simulink model "chan_snap_v3"  (R2012b)
settings: Solver=ode45  StartTime=0.0  StopTime=10000  RelTol=1e-3
undefined symbols (not defined in the file): pfb_coeff_gen_calc, xlipgetpartsetting
libraries: xbsIndex_r4 x7452, casper_library_misc x131, casper_library_flow_control x107, casper_library_delays x40, xps_library x8
(part 3 of 84)

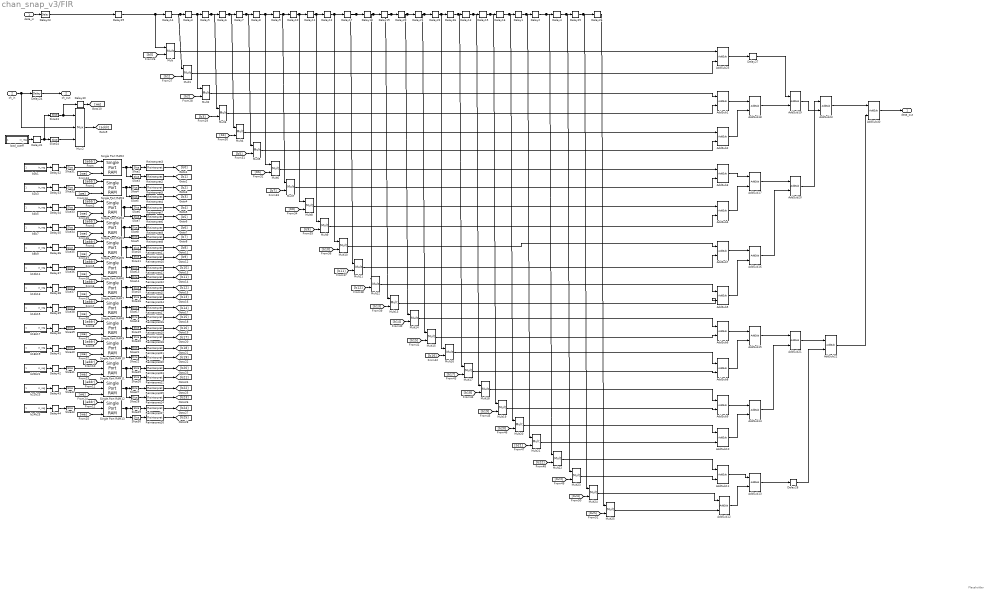
== system chan_snap_v3/FIR ==
  note: Placeholder
  data_in : Inport
  ch_in : Inport  Port=2
  AddSub{1..23,25} (24 alike) : xbsIndex_r4/AddSub  mode=Addition  use_carryin=off  use_carryout=off  en=off  latency=3  precision=Full  arith_type="Signed  (2's comp)"  n_bits=16  bin_pt=15  quantization=Truncate  overflow=Wrap  dbl_ovrd=off  use_behavioral_HDL=off  hw_selection=DSP48  pipelined=on  block_type=addsub
  AddSub40 : xbsIndex_r4/AddSub  mode=Addition  use_carryin=off  use_carryout=off  en=off  latency=3  precision=User Defined  arith_type="Signed  (2's comp)"  n_bits=12  bin_pt=9  quantization=Truncate  overflow=Wrap  dbl_ovrd=off  use_behavioral_HDL=off  hw_selection=DSP48  pipelined=on  block_type=addsub
  Delay{1..22,25..26,46} (25 alike) : xbsIndex_r4/Delay  rst=off  infoeditControl=Selection of Reset will increase slice count due to use of real FFs and instead of SRLs  en=off  latency=256  dbl_ovrd=off  reg_retiming=off  block_type=delay
      settings: block_version=11.4
  Delay{23,30..44} (16 alike) : xbsIndex_r4/Delay  rst=off  infoeditControl=Selection of Reset will increase slice count due to use of real FFs and instead of SRLs  en=off  latency=1  dbl_ovrd=off  reg_retiming=off  block_type=delay
      settings: block_version=11.4
  Delay24 : xbsIndex_r4/Delay  rst=off  infoeditControl=Selection of Reset will increase slice count due to use of real FFs and instead of SRLs  en=off  latency=24  dbl_ovrd=off  reg_retiming=off  block_type=delay
      settings: block_version=11.4
  Delay27 : xbsIndex_r4/Delay  rst=off  infoeditControl=Selection of Reset will increase slice count due to use of real FFs and instead of SRLs  en=off  latency=3  dbl_ovrd=off  reg_retiming=off  block_type=delay
      settings: block_version=11.4
  Delay28 : xbsIndex_r4/Delay  rst=off  infoeditControl=Selection of Reset will increase slice count due to use of real FFs and instead of SRLs  en=off  latency=3  dbl_ovrd=off  reg_retiming=off  block_type=delay
      settings: block_version=11.4
  Delay29 : xbsIndex_r4/Delay  rst=off  infoeditControl=Selection of Reset will increase slice count due to use of real FFs and instead of SRLs  en=off  latency=3  dbl_ovrd=off  reg_retiming=off  block_type=delay
      settings: block_version=11.4
  Mult{,1..25} (26 alike) : xbsIndex_r4/Mult  precision=Full  arith_type="Signed  (2's comp)"  n_bits=16  bin_pt=14  quantization=Truncate  overflow=Wrap  en=off  latency=5  dbl_ovrd=off  use_behavioral_HDL=off  opt=Speed  use_embedded=on  optimum_pipeline=on  pipeline=on  use_rpm=on  placement_style=Triangular  block_type=mult
      settings: block_version=11.4
  Mux2 : xbsIndex_r4/Mux  inputs=2  en=off  latency=1  precision=Full  arith_type=Unsigned  n_bits=16  bin_pt=14  quantization=Truncate  overflow=Wrap  dbl_ovrd=off  block_type=mux
      settings: block_version=11.4
  Reinterpret{2..27} (26 alike) : xbsIndex_r4/Reinterpret  force_arith_type=on  arith_type="Signed  (2's comp)"  force_bin_pt=on  bin_pt=11  block_type=reinterpret
      settings: infoedit="Changes signal type without altering the binary representation.   You can changed the signal between signed and unsigned, and relocate the binary point.<br><br>Hardware notes: In hardware this block costs nothing.<br><br>Example:  Suppose the input is 6 bits wide, signed, with 2 fractional bits, and the output is forced to unsigned with 0 fractional bits.  Then an input of -2.0 (1110.00 in binary 2's complement) becomes an output of 56 (111000 in binary)."
  Single Port RAM1 : xbsIndex_r4/Single Port RAM  depth=256  initVector=[97453145 97453145 97453145 97453145 97453145 97453145 97453145 97453145 97453145 97453145]  distributed_mem=Block RAM  write_mode=No Read On Write  rst=off  init_reg=0  en=off  latency=3  dbl_ovrd=off  optimize=Speed  block_type=spram
  Single Port RAM10 : xbsIndex_r4/Single Port RAM  depth=256  initVector=[72943055 72943055 72943055 72943055 72943055 72943055 72943055 72943055 72943055 72943055 ]  distributed_mem=Block RAM  write_mode=No Read On Write  rst=off  init_reg=0  en=off  latency=3  dbl_ovrd=off  optimize=Speed  block_type=spram
  Single Port RAM11 : xbsIndex_r4/Single Port RAM  depth=256  initVector=[31523587 31523587 31523587 31523587 31523587 31523587 31523587 31523587 31523587 31523587 ]  distributed_mem=Block RAM  write_mode=No Read On Write  rst=off  init_reg=0  en=off  latency=3  dbl_ovrd=off  optimize=Speed  block_type=spram
  Single Port RAM12 : xbsIndex_r4/Single Port RAM  depth=256  initVector=[6947073 6947073 6947073 6947073 6947073 6947073 6947073 6947073 6947073 6947073 ]  distributed_mem=Block RAM  write_mode=No Read On Write  rst=off  init_reg=0  en=off  latency=3  dbl_ovrd=off  optimize=Speed  block_type=spram
  Single Port RAM13 : xbsIndex_r4/Single Port RAM  depth=256  initVector=[24 24 24 24 24 24 24 24 24 24 ]  distributed_mem=Block RAM  write_mode=No Read On Write  rst=off  init_reg=0  en=off  latency=3  dbl_ovrd=off  optimize=Speed  block_type=spram
  Single Port RAM2 : xbsIndex_r4/Single Port RAM  depth=256  initVector=[1572864 1572864 1572864 1572864 1572864 1572864 1572864 1572864 1572864 1572864]  distributed_mem=Block RAM  write_mode=No Read On Write  rst=off  init_reg=0  en=off  latency=3  dbl_ovrd=off  optimize=Speed  block_type=spram
  Single Port RAM3 : xbsIndex_r4/Single Port RAM  depth=256  initVector=[16842858 16842858 16842858 16842858 16842858 16842858 16842858 16842858 16842858 16842858]  distributed_mem=Block RAM  write_mode=No Read On Write  rst=off  init_reg=0  en=off  latency=3  dbl_ovrd=off  optimize=Speed  block_type=spram
  Single Port RAM4 : xbsIndex_r4/Single Port RAM  depth=256  initVector=[50528737 50528737 50528737 50528737 50528737 50528737 50528737 50528737 50528737 50528737]  distributed_mem=Block RAM  write_mode=No Read On Write  rst=off  init_reg=0  en=off  latency=3  dbl_ovrd=off  optimize=Speed  block_type=spram
  Single Port RAM5 : xbsIndex_r4/Single Port RAM  depth=256  initVector=[145098568 145098568 145098568 145098568 145098568 145098568 145098568 145098568 145098568 145098568]  distributed_mem=Block RAM  write_mode=No Read On Write  rst=off  init_reg=0  en=off  latency=3  dbl_ovrd=off  optimize=Speed  block_type=spram
  Single Port RAM6 : xbsIndex_r4/Single Port RAM  depth=256  initVector=[178325964 178325964 178325964 178325964 178325964 178325964 178325964 178325964 178325964 178325964]  distributed_mem=Block RAM  write_mode=No Read On Write  rst=off  init_reg=0  en=off  latency=3  dbl_ovrd=off  optimize=Speed  block_type=spram
  Single Port RAM7 : xbsIndex_r4/Single Port RAM  depth=256  initVector=[185600784 185600784 185600784 185600784 185600784 185600784 185600784 185600784 185600784 185600784]  distributed_mem=Block RAM  write_mode=No Read On Write  rst=off  init_reg=0  en=off  latency=3  dbl_ovrd=off  optimize=Speed  block_type=spram
  Single Port RAM8 : xbsIndex_r4/Single Port RAM  depth=256  initVector=[164367009 164367009 164367009 164367009 164367009 164367009 164367009 164367009 164367009 164367009 ]  distributed_mem=Block RAM  write_mode=No Read On Write  rst=off  init_reg=0  en=off  latency=3  dbl_ovrd=off  optimize=Speed  block_type=spram
  Single Port RAM9 : xbsIndex_r4/Single Port RAM  depth=256  initVector=[122161318 122161318 122161318 122161318 122161318 122161318 122161318 122161318 122161318 122161318 ]  distributed_mem=Block RAM  write_mode=No Read On Write  rst=off  init_reg=0  en=off  latency=3  dbl_ovrd=off  optimize=Speed  block_type=spram
  Slice{2,4,6,8,10,13,15,17,19,21,25,27,29} (13 alike) : xbsIndex_r4/Slice  nbits=12  boolean_output=off  mode=Lower Bit Location + Width  bit1=0  base1=MSB of Input  bit0=0  base0=LSB of Input  dbl_ovrd=off  block_type=slice
      settings: block_version=10.1.3
  Slice{3,5,7,9,11,14,16,18,20,22,26,28,30} (13 alike) : xbsIndex_r4/Slice  nbits=12  boolean_output=off  mode=Lower Bit Location + Width  bit1=0  base1=MSB of Input  bit0=12  base0=LSB of Input  dbl_ovrd=off  block_type=slice
      settings: block_version=10.1.3
  Slice23 : xbsIndex_r4/Slice  nbits=16  boolean_output=on  mode=Lower Bit Location + Width  bit1=0  base1=MSB of Input  bit0=0  base0=LSB of Input  dbl_ovrd=off  block_type=slice
      settings: block_version=10.1.3
  Slice24 : xbsIndex_r4/Slice  nbits=8  boolean_output=off  mode=Lower Bit Location + Width  bit1=0  base1=MSB of Input  bit0=1  base0=LSB of Input  dbl_ovrd=off  block_type=slice
      settings: block_version=10.1.3
  Slice{31..43} (13 alike) : xbsIndex_r4/Slice  nbits=24  boolean_output=off  mode=Lower Bit Location + Width  bit1=0  base1=MSB of Input  bit0=0  base0=LSB of Input  dbl_ovrd=off  block_type=slice
      settings: block_version=10.1.3
  b0b1 : Subsystem  Tag=xps:sw_reg  AncestorBlock=xps_library/software register  mask{numios=1, io_dir=From Processor, io_delay=0, sample_period=1, name1=reg, bitwidth1=32, arith_type1=Unsigned, bin_pt1=0}
      mask prompts: numios "Num I/Os"; io_dir "I/O direction"; io_delay "I/O delay"; sample_period "Sample period"; name1 "Name"; bitwidth1 "Bitwidth"; arith_type1 "Type"; bin_pt1 "Binary pt"
      mask init:
      | swreg_init(gcb);
      mask Callback numios: t = timer('StartDelay', 0.1); t.TimerFcn = {@swreg_cb, gcb}; start(t);
      mask TypeOptions io_dir: To Processor | From Processor
      mask Callback io_dir:
      | a = get_param(gcb, 'MaskEnables');
      | if strcmp(get_param(gcb, 'io_dir'), 'To Processor'),
      | a(4) = {'off'};
      | else
      | a(4) = {'on'};
      | end
      | set_param(gcb, 'MaskEnables', a);
      mask TypeOptions arith_type1: Unsigned | Signed  (2's comp) | Boolean
      mask Callback arith_type1:
      | a = get_param(gcb, 'MaskEnables');
      | if strcmp(get_param(gcb, 'arith_type1'), 'Boolean'),
      | set_param(gcb, 'bitwidth1', '1');
      | set_param(gcb, 'bin_pt1', '0');
      | a(6) = {'off'};
      | a(8) = {'off'};
      | else
      | a(6) = {'on'};
      | a(8) = {'on'};
      | end
      | set_param(gcb, 'MaskEnables', a);
  b10b11 : Subsystem  Tag=xps:sw_reg  AncestorBlock=xps_library/software register  mask{numios=1, io_dir=From Processor, io_delay=0, sample_period=1, name1=reg, bitwidth1=32, arith_type1=Unsigned, bin_pt1=0}
      mask prompts: numios "Num I/Os"; io_dir "I/O direction"; io_delay "I/O delay"; sample_period "Sample period"; name1 "Name"; bitwidth1 "Bitwidth"; arith_type1 "Type"; bin_pt1 "Binary pt"
      mask init:
      | swreg_init(gcb);
      mask Callback numios: t = timer('StartDelay', 0.1); t.TimerFcn = {@swreg_cb, gcb}; start(t);
      mask TypeOptions io_dir: To Processor | From Processor
      mask Callback io_dir:
      | a = get_param(gcb, 'MaskEnables');
      | if strcmp(get_param(gcb, 'io_dir'), 'To Processor'),
      | a(4) = {'off'};
      | else
      | a(4) = {'on'};
      | end
      | set_param(gcb, 'MaskEnables', a);
      mask TypeOptions arith_type1: Unsigned | Signed  (2's comp) | Boolean
      mask Callback arith_type1:
      | a = get_param(gcb, 'MaskEnables');
      | if strcmp(get_param(gcb, 'arith_type1'), 'Boolean'),
      | set_param(gcb, 'bitwidth1', '1');
      | set_param(gcb, 'bin_pt1', '0');
      | a(6) = {'off'};
      | a(8) = {'off'};
      | else
      | a(6) = {'on'};
      | a(8) = {'on'};
      | end
      | set_param(gcb, 'MaskEnables', a);
  b12b13 : Subsystem  Tag=xps:sw_reg  AncestorBlock=xps_library/software register  mask{numios=1, io_dir=From Processor, io_delay=0, sample_period=1, name1=reg, bitwidth1=32, arith_type1=Unsigned, bin_pt1=0}
      mask prompts: numios "Num I/Os"; io_dir "I/O direction"; io_delay "I/O delay"; sample_period "Sample period"; name1 "Name"; bitwidth1 "Bitwidth"; arith_type1 "Type"; bin_pt1 "Binary pt"
      mask init:
      | swreg_init(gcb);
      mask Callback numios: t = timer('StartDelay', 0.1); t.TimerFcn = {@swreg_cb, gcb}; start(t);
      mask TypeOptions io_dir: To Processor | From Processor
      mask Callback io_dir:
      | a = get_param(gcb, 'MaskEnables');
      | if strcmp(get_param(gcb, 'io_dir'), 'To Processor'),
      | a(4) = {'off'};
      | else
      | a(4) = {'on'};
      | end
      | set_param(gcb, 'MaskEnables', a);
      mask TypeOptions arith_type1: Unsigned | Signed  (2's comp) | Boolean
      mask Callback arith_type1:
      | a = get_param(gcb, 'MaskEnables');
      | if strcmp(get_param(gcb, 'arith_type1'), 'Boolean'),
      | set_param(gcb, 'bitwidth1', '1');
      | set_param(gcb, 'bin_pt1', '0');
      | a(6) = {'off'};
      | a(8) = {'off'};
      | else
      | a(6) = {'on'};
      | a(8) = {'on'};
      | end
      | set_param(gcb, 'MaskEnables', a);
  b14b15 : Subsystem  Tag=xps:sw_reg  AncestorBlock=xps_library/software register  mask{numios=1, io_dir=From Processor, io_delay=0, sample_period=1, name1=reg, bitwidth1=32, arith_type1=Unsigned, bin_pt1=0}
      mask prompts: numios "Num I/Os"; io_dir "I/O direction"; io_delay "I/O delay"; sample_period "Sample period"; name1 "Name"; bitwidth1 "Bitwidth"; arith_type1 "Type"; bin_pt1 "Binary pt"
      mask init:
      | swreg_init(gcb);
      mask Callback numios: t = timer('StartDelay', 0.1); t.TimerFcn = {@swreg_cb, gcb}; start(t);
      mask TypeOptions io_dir: To Processor | From Processor
      mask Callback io_dir:
      | a = get_param(gcb, 'MaskEnables');
      | if strcmp(get_param(gcb, 'io_dir'), 'To Processor'),
      | a(4) = {'off'};
      | else
      | a(4) = {'on'};
      | end
      | set_param(gcb, 'MaskEnables', a);
      mask TypeOptions arith_type1: Unsigned | Signed  (2's comp) | Boolean
      mask Callback arith_type1:
      | a = get_param(gcb, 'MaskEnables');
      | if strcmp(get_param(gcb, 'arith_type1'), 'Boolean'),
      | set_param(gcb, 'bitwidth1', '1');
      | set_param(gcb, 'bin_pt1', '0');
      | a(6) = {'off'};
      | a(8) = {'off'};
      | else
      | a(6) = {'on'};
      | a(8) = {'on'};
      | end
      | set_param(gcb, 'MaskEnables', a);
  b16b17 : Subsystem  Tag=xps:sw_reg  AncestorBlock=xps_library/software register  mask{numios=1, io_dir=From Processor, io_delay=0, sample_period=1, name1=reg, bitwidth1=32, arith_type1=Unsigned, bin_pt1=0}
      mask prompts: numios "Num I/Os"; io_dir "I/O direction"; io_delay "I/O delay"; sample_period "Sample period"; name1 "Name"; bitwidth1 "Bitwidth"; arith_type1 "Type"; bin_pt1 "Binary pt"
      mask init:
      | swreg_init(gcb);
      mask Callback numios: t = timer('StartDelay', 0.1); t.TimerFcn = {@swreg_cb, gcb}; start(t);
      mask TypeOptions io_dir: To Processor | From Processor
      mask Callback io_dir:
      | a = get_param(gcb, 'MaskEnables');
      | if strcmp(get_param(gcb, 'io_dir'), 'To Processor'),
      | a(4) = {'off'};
      | else
      | a(4) = {'on'};
      | end
      | set_param(gcb, 'MaskEnables', a);
      mask TypeOptions arith_type1: Unsigned | Signed  (2's comp) | Boolean
      mask Callback arith_type1:
      | a = get_param(gcb, 'MaskEnables');
      | if strcmp(get_param(gcb, 'arith_type1'), 'Boolean'),
      | set_param(gcb, 'bitwidth1', '1');
      | set_param(gcb, 'bin_pt1', '0');
      | a(6) = {'off'};
      | a(8) = {'off'};
      | else
      | a(6) = {'on'};
      | a(8) = {'on'};
      | end
      | set_param(gcb, 'MaskEnables', a);
  b18b19 : Subsystem  Tag=xps:sw_reg  AncestorBlock=xps_library/software register  mask{numios=1, io_dir=From Processor, io_delay=0, sample_period=1, name1=reg, bitwidth1=32, arith_type1=Unsigned, bin_pt1=0}
      mask prompts: numios "Num I/Os"; io_dir "I/O direction"; io_delay "I/O delay"; sample_period "Sample period"; name1 "Name"; bitwidth1 "Bitwidth"; arith_type1 "Type"; bin_pt1 "Binary pt"
      mask init:
      | swreg_init(gcb);
      mask Callback numios: t = timer('StartDelay', 0.1); t.TimerFcn = {@swreg_cb, gcb}; start(t);
      mask TypeOptions io_dir: To Processor | From Processor
      mask Callback io_dir:
      | a = get_param(gcb, 'MaskEnables');
      | if strcmp(get_param(gcb, 'io_dir'), 'To Processor'),
      | a(4) = {'off'};
      | else
      | a(4) = {'on'};
      | end
      | set_param(gcb, 'MaskEnables', a);
      mask TypeOptions arith_type1: Unsigned | Signed  (2's comp) | Boolean
      mask Callback arith_type1:
      | a = get_param(gcb, 'MaskEnables');
      | if strcmp(get_param(gcb, 'arith_type1'), 'Boolean'),
      | set_param(gcb, 'bitwidth1', '1');
      | set_param(gcb, 'bin_pt1', '0');
      | a(6) = {'off'};
      | a(8) = {'off'};
      | else
      | a(6) = {'on'};
      | a(8) = {'on'};
      | end
      | set_param(gcb, 'MaskEnables', a);
  b20b21 : Subsystem  Tag=xps:sw_reg  AncestorBlock=xps_library/software register  mask{numios=1, io_dir=From Processor, io_delay=0, sample_period=1, name1=reg, bitwidth1=32, arith_type1=Unsigned, bin_pt1=0}
      mask prompts: numios "Num I/Os"; io_dir "I/O direction"; io_delay "I/O delay"; sample_period "Sample period"; name1 "Name"; bitwidth1 "Bitwidth"; arith_type1 "Type"; bin_pt1 "Binary pt"
      mask init:
      | swreg_init(gcb);
      mask Callback numios: t = timer('StartDelay', 0.1); t.TimerFcn = {@swreg_cb, gcb}; start(t);
      mask TypeOptions io_dir: To Processor | From Processor
      mask Callback io_dir:
      | a = get_param(gcb, 'MaskEnables');
      | if strcmp(get_param(gcb, 'io_dir'), 'To Processor'),
      | a(4) = {'off'};
      | else
      | a(4) = {'on'};
      | end
      | set_param(gcb, 'MaskEnables', a);
      mask TypeOptions arith_type1: Unsigned | Signed  (2's comp) | Boolean
      mask Callback arith_type1:
      | a = get_param(gcb, 'MaskEnables');
      | if strcmp(get_param(gcb, 'arith_type1'), 'Boolean'),
      | set_param(gcb, 'bitwidth1', '1');
      | set_param(gcb, 'bin_pt1', '0');
      | a(6) = {'off'};
      | a(8) = {'off'};
      | else
      | a(6) = {'on'};
      | a(8) = {'on'};
      | end
      | set_param(gcb, 'MaskEnables', a);
  b22b23 : Subsystem  Tag=xps:sw_reg  AncestorBlock=xps_library/software register  mask{numios=1, io_dir=From Processor, io_delay=0, sample_period=1, name1=reg, bitwidth1=32, arith_type1=Unsigned, bin_pt1=0}
      mask prompts: numios "Num I/Os"; io_dir "I/O direction"; io_delay "I/O delay"; sample_period "Sample period"; name1 "Name"; bitwidth1 "Bitwidth"; arith_type1 "Type"; bin_pt1 "Binary pt"
      mask init:
      | swreg_init(gcb);
      mask Callback numios: t = timer('StartDelay', 0.1); t.TimerFcn = {@swreg_cb, gcb}; start(t);
      mask TypeOptions io_dir: To Processor | From Processor
      mask Callback io_dir:
      | a = get_param(gcb, 'MaskEnables');
      | if strcmp(get_param(gcb, 'io_dir'), 'To Processor'),
      | a(4) = {'off'};
      | else
      | a(4) = {'on'};
      | end
      | set_param(gcb, 'MaskEnables', a);
      mask TypeOptions arith_type1: Unsigned | Signed  (2's comp) | Boolean
      mask Callback arith_type1:
      | a = get_param(gcb, 'MaskEnables');
      | if strcmp(get_param(gcb, 'arith_type1'), 'Boolean'),
      | set_param(gcb, 'bitwidth1', '1');
      | set_param(gcb, 'bin_pt1', '0');
      | a(6) = {'off'};
      | a(8) = {'off'};
      | else
      | a(6) = {'on'};
      | a(8) = {'on'};
      | end
      | set_param(gcb, 'MaskEnables', a);
  b24b25 : Subsystem  Tag=xps:sw_reg  AncestorBlock=xps_library/software register  mask{numios=1, io_dir=From Processor, io_delay=0, sample_period=1, name1=reg, bitwidth1=32, arith_type1=Unsigned, bin_pt1=0}
      mask prompts: numios "Num I/Os"; io_dir "I/O direction"; io_delay "I/O delay"; sample_period "Sample period"; name1 "Name"; bitwidth1 "Bitwidth"; arith_type1 "Type"; bin_pt1 "Binary pt"
      mask init:
      | swreg_init(gcb);
      mask Callback numios: t = timer('StartDelay', 0.1); t.TimerFcn = {@swreg_cb, gcb}; start(t);
      mask TypeOptions io_dir: To Processor | From Processor
      mask Callback io_dir:
      | a = get_param(gcb, 'MaskEnables');
      | if strcmp(get_param(gcb, 'io_dir'), 'To Processor'),
      | a(4) = {'off'};
      | else
      | a(4) = {'on'};
      | end
      | set_param(gcb, 'MaskEnables', a);
      mask TypeOptions arith_type1: Unsigned | Signed  (2's comp) | Boolean
      mask Callback arith_type1:
      | a = get_param(gcb, 'MaskEnables');
      | if strcmp(get_param(gcb, 'arith_type1'), 'Boolean'),
      | set_param(gcb, 'bitwidth1', '1');
      | set_param(gcb, 'bin_pt1', '0');
      | a(6) = {'off'};
      | a(8) = {'off'};
      | else
      | a(6) = {'on'};
      | a(8) = {'on'};
      | end
      | set_param(gcb, 'MaskEnables', a);
  b2b3 : Subsystem  Tag=xps:sw_reg  AncestorBlock=xps_library/software register  mask{numios=1, io_dir=From Processor, io_delay=0, sample_period=1, name1=reg, bitwidth1=32, arith_type1=Unsigned, bin_pt1=0}
      mask prompts: numios "Num I/Os"; io_dir "I/O direction"; io_delay "I/O delay"; sample_period "Sample period"; name1 "Name"; bitwidth1 "Bitwidth"; arith_type1 "Type"; bin_pt1 "Binary pt"
      mask init:
      | swreg_init(gcb);
      mask Callback numios: t = timer('StartDelay', 0.1); t.TimerFcn = {@swreg_cb, gcb}; start(t);
      mask TypeOptions io_dir: To Processor | From Processor
      mask Callback io_dir:
      | a = get_param(gcb, 'MaskEnables');
      | if strcmp(get_param(gcb, 'io_dir'), 'To Processor'),
      | a(4) = {'off'};
      | else
      | a(4) = {'on'};
      | end
      | set_param(gcb, 'MaskEnables', a);
      mask TypeOptions arith_type1: Unsigned | Signed  (2's comp) | Boolean
      mask Callback arith_type1:
      | a = get_param(gcb, 'MaskEnables');
      | if strcmp(get_param(gcb, 'arith_type1'), 'Boolean'),
      | set_param(gcb, 'bitwidth1', '1');
      | set_param(gcb, 'bin_pt1', '0');
      | a(6) = {'off'};
      | a(8) = {'off'};
      | else
      | a(6) = {'on'};
      | a(8) = {'on'};
      | end
      | set_param(gcb, 'MaskEnables', a);
  b4b5 : Subsystem  Tag=xps:sw_reg  AncestorBlock=xps_library/software register  mask{numios=1, io_dir=From Processor, io_delay=0, sample_period=1, name1=reg, bitwidth1=32, arith_type1=Unsigned, bin_pt1=0}
      mask prompts: numios "Num I/Os"; io_dir "I/O direction"; io_delay "I/O delay"; sample_period "Sample period"; name1 "Name"; bitwidth1 "Bitwidth"; arith_type1 "Type"; bin_pt1 "Binary pt"
      mask init:
      | swreg_init(gcb);
      mask Callback numios: t = timer('StartDelay', 0.1); t.TimerFcn = {@swreg_cb, gcb}; start(t);
      mask TypeOptions io_dir: To Processor | From Processor
      mask Callback io_dir:
      | a = get_param(gcb, 'MaskEnables');
      | if strcmp(get_param(gcb, 'io_dir'), 'To Processor'),
      | a(4) = {'off'};
      | else
      | a(4) = {'on'};
      | end
      | set_param(gcb, 'MaskEnables', a);
      mask TypeOptions arith_type1: Unsigned | Signed  (2's comp) | Boolean
      mask Callback arith_type1:
      | a = get_param(gcb, 'MaskEnables');
      | if strcmp(get_param(gcb, 'arith_type1'), 'Boolean'),
      | set_param(gcb, 'bitwidth1', '1');
      | set_param(gcb, 'bin_pt1', '0');
      | a(6) = {'off'};
      | a(8) = {'off'};
      | else
      | a(6) = {'on'};
      | a(8) = {'on'};
      | end
      | set_param(gcb, 'MaskEnables', a);
  b6b7 : Subsystem  Tag=xps:sw_reg  AncestorBlock=xps_library/software register  mask{numios=1, io_dir=From Processor, io_delay=0, sample_period=1, name1=reg, bitwidth1=32, arith_type1=Unsigned, bin_pt1=0}
      mask prompts: numios "Num I/Os"; io_dir "I/O direction"; io_delay "I/O delay"; sample_period "Sample period"; name1 "Name"; bitwidth1 "Bitwidth"; arith_type1 "Type"; bin_pt1 "Binary pt"
      mask init:
      | swreg_init(gcb);
      mask Callback numios: t = timer('StartDelay', 0.1); t.TimerFcn = {@swreg_cb, gcb}; start(t);
      mask TypeOptions io_dir: To Processor | From Processor
      mask Callback io_dir:
      | a = get_param(gcb, 'MaskEnables');
      | if strcmp(get_param(gcb, 'io_dir'), 'To Processor'),
      | a(4) = {'off'};
      | else
      | a(4) = {'on'};
      | end
      | set_param(gcb, 'MaskEnables', a);
      mask TypeOptions arith_type1: Unsigned | Signed  (2's comp) | Boolean
      mask Callback arith_type1:
      | a = get_param(gcb, 'MaskEnables');
      | if strcmp(get_param(gcb, 'arith_type1'), 'Boolean'),
      | set_param(gcb, 'bitwidth1', '1');
      | set_param(gcb, 'bin_pt1', '0');
      | a(6) = {'off'};
      | a(8) = {'off'};
      | else
      | a(6) = {'on'};
      | a(8) = {'on'};
      | end
      | set_param(gcb, 'MaskEnables', a);
  b8b9 : Subsystem  Tag=xps:sw_reg  AncestorBlock=xps_library/software register  mask{numios=1, io_dir=From Processor, io_delay=0, sample_period=1, name1=reg, bitwidth1=32, arith_type1=Unsigned, bin_pt1=0}
      mask prompts: numios "Num I/Os"; io_dir "I/O direction"; io_delay "I/O delay"; sample_period "Sample period"; name1 "Name"; bitwidth1 "Bitwidth"; arith_type1 "Type"; bin_pt1 "Binary pt"
      mask init:
      | swreg_init(gcb);
      mask Callback numios: t = timer('StartDelay', 0.1); t.TimerFcn = {@swreg_cb, gcb}; start(t);
      mask TypeOptions io_dir: To Processor | From Processor
      mask Callback io_dir:
      | a = get_param(gcb, 'MaskEnables');
      | if strcmp(get_param(gcb, 'io_dir'), 'To Processor'),
      | a(4) = {'off'};
      | else
      | a(4) = {'on'};
      | end
      | set_param(gcb, 'MaskEnables', a);
      mask TypeOptions arith_type1: Unsigned | Signed  (2's comp) | Boolean
      mask Callback arith_type1:
      | a = get_param(gcb, 'MaskEnables');
      | if strcmp(get_param(gcb, 'arith_type1'), 'Boolean'),
      | set_param(gcb, 'bitwidth1', '1');
      | set_param(gcb, 'bin_pt1', '0');
      | a(6) = {'off'};
      | a(8) = {'off'};
      | else
      | a(6) = {'on'};
      | a(8) = {'on'};
      | end
      | set_param(gcb, 'MaskEnables', a);
  load_coeff : Subsystem  Tag=xps:sw_reg  AncestorBlock=xps_library/software register  mask{numios=1, io_dir=From Processor, io_delay=0, sample_period=1, name1=reg, bitwidth1=32, arith_type1=Unsigned, bin_pt1=0}
      mask prompts: numios "Num I/Os"; io_dir "I/O direction"; io_delay "I/O delay"; sample_period "Sample period"; name1 "Name"; bitwidth1 "Bitwidth"; arith_type1 "Type"; bin_pt1 "Binary pt"
      mask init:
      | swreg_init(gcb);
      mask Callback numios: t = timer('StartDelay', 0.1); t.TimerFcn = {@swreg_cb, gcb}; start(t);
      mask TypeOptions io_dir: To Processor | From Processor
      mask Callback io_dir:
      | a = get_param(gcb, 'MaskEnables');
      | if strcmp(get_param(gcb, 'io_dir'), 'To Processor'),
      | a(4) = {'off'};
      | else
      | a(4) = {'on'};
      | end
      | set_param(gcb, 'MaskEnables', a);
      mask TypeOptions arith_type1: Unsigned | Signed  (2's comp) | Boolean
      mask Callback arith_type1:
      | a = get_param(gcb, 'MaskEnables');
      | if strcmp(get_param(gcb, 'arith_type1'), 'Boolean'),
      | set_param(gcb, 'bitwidth1', '1');
      | set_param(gcb, 'bin_pt1', '0');
      | a(6) = {'off'};
      | a(8) = {'off'};
      | else
      | a(6) = {'on'};
      | a(8) = {'on'};
      | end
      | set_param(gcb, 'MaskEnables', a);
  data_out : Outport
  ch_out : Outport  Port=2
  wires:
  data_in/1 -> Delay23/1
  ch_in/1 -> Mux2/2, Delay24/1
  Delay24/1 -> ch_out/1
  load_coeff/1(in_reg) -> Delay31/1
  Slice23/1 -> Mux2/1, Delay30/1
  Slice24/1 -> Mux2/3
  b0b1/1(in_reg) -> Delay32/1
  b2b3/1(in_reg) -> Delay33/1
  b4b5/1(in_reg) -> Delay34/1
  b6b7/1(in_reg) -> Delay35/1
  b8b9/1(in_reg) -> Delay36/1
  b10b11/1(in_reg) -> Delay37/1
  b12b13/1(in_reg) -> Delay38/1
  b14b15/1(in_reg) -> Delay39/1
  b16b17/1(in_reg) -> Delay40/1
  b18b19/1(in_reg) -> Delay41/1
  b20b21/1(in_reg) -> Delay42/1
  b22b23/1(in_reg) -> Delay43/1
  b24b25/1(in_reg) -> Delay44/1
  Single Port RAM2/1 -> Slice2/1, Slice3/1
  Slice2/1 -> Reinterpret3/1
  Slice3/1 -> Reinterpret2/1
  Single Port RAM3/1 -> Slice4/1, Slice5/1
  Slice4/1 -> Reinterpret5/1
  Slice5/1 -> Reinterpret4/1
  Single Port RAM4/1 -> Slice6/1, Slice7/1
  Slice6/1 -> Reinterpret7/1
  Slice7/1 -> Reinterpret6/1
  Single Port RAM1/1 -> Slice9/1, Slice8/1
  Slice8/1 -> Reinterpret9/1
  Slice9/1 -> Reinterpret8/1
  Single Port RAM5/1 -> Slice10/1, Slice11/1
  Slice10/1 -> Reinterpret11/1
  Slice11/1 -> Reinterpret10/1
  Single Port RAM6/1 -> Slice14/1, Slice13/1
  Slice13/1 -> Reinterpret13/1
  Slice14/1 -> Reinterpret12/1
  Single Port RAM7/1 -> Slice16/1, Slice15/1
  Slice15/1 -> Reinterpret15/1
  Slice16/1 -> Reinterpret14/1
  Single Port RAM8/1 -> Slice17/1, Slice18/1
  Slice17/1 -> Reinterpret17/1
  Slice18/1 -> Reinterpret16/1
  Single Port RAM9/1 -> Slice19/1, Slice20/1
  Slice19/1 -> Reinterpret19/1
  Slice20/1 -> Reinterpret18/1
  Single Port RAM10/1 -> Slice22/1, Slice21/1
  Slice21/1 -> Reinterpret21/1
  Slice22/1 -> Reinterpret20/1
  Single Port RAM11/1 -> Slice26/1, Slice25/1
  Slice25/1 -> Reinterpret23/1
  Slice26/1 -> Reinterpret22/1
  Single Port RAM12/1 -> Slice27/1, Slice28/1
  Slice27/1 -> Reinterpret25/1
  Slice28/1 -> Reinterpret24/1
  Single Port RAM13/1 -> Slice30/1, Slice29/1
  Slice29/1 -> Reinterpret27/1
  Slice30/1 -> Reinterpret26/1
  Mux2/1 -> [addr]
  [addr] -> Single Port RAM2/1
  [addr] -> Single Port RAM3/1
  [addr] -> Single Port RAM4/1
  [addr] -> Single Port RAM1/1
  [addr] -> Single Port RAM5/1
  [addr] -> Single Port RAM6/1
  [addr] -> Single Port RAM7/1
  [addr] -> Single Port RAM9/1
  [addr] -> Single Port RAM8/1
  [addr] -> Single Port RAM10/1
  [addr] -> Single Port RAM11/1
  [addr] -> Single Port RAM12/1
  [addr] -> Single Port RAM13/1
  [we] -> Single Port RAM2/3
  [we] -> Single Port RAM3/3
  [we] -> Single Port RAM4/3
  [we] -> Single Port RAM1/3
  [we] -> Single Port RAM5/3
  [we] -> Single Port RAM6/3
  [we] -> Single Port RAM7/3
  [we] -> Single Port RAM8/3
  [we] -> Single Port RAM9/3
  [we] -> Single Port RAM10/3
  [we] -> Single Port RAM11/3
  [we] -> Single Port RAM12/3
  [we] -> Single Port RAM13/3
  Delay14/1 -> Mult1/1, Delay3/1
  Delay23/1 -> Delay29/1
  [b4] -> Mult4/2
  [b5] -> Mult5/2
  [b6] -> Mult6/2
  [b7] -> Mult7/2
  [b8] -> Mult8/2
  [b9] -> Mult9/2
  [b10] -> Mult10/2
  [b11] -> Mult11/2
  [b12] -> Mult12/2
  [b13] -> Mult13/2
  [b14] -> Mult14/2
  [b15] -> Mult15/2
  [b16] -> Mult16/2
  [b17] -> Mult17/2
  [b18] -> Mult18/2
  [b19] -> Mult19/2
  [b20] -> Mult20/2
  [b21] -> Mult21/2
  [b22] -> Mult22/2
  [b23] -> Mult23/2
  [b24] -> Mult24/2
  [b25] -> Mult25/2
  Mult24/1 -> AddSub12/1
  Reinterpret3/1 -> [b0]
  Reinterpret2/1 -> [b1]
  Reinterpret5/1 -> [b2]
  Reinterpret4/1 -> [b3]
  Reinterpret7/1 -> [b4]
  Reinterpret6/1 -> [b5]
  Reinterpret9/1 -> [b6]
  Reinterpret8/1 -> [b7]
  Reinterpret11/1 -> [b8]
  Reinterpret10/1 -> [b9]
  Reinterpret13/1 -> [b10]
  Reinterpret12/1 -> [b11]
  Reinterpret15/1 -> [b12]
  Reinterpret14/1 -> [b13]
  Reinterpret17/1 -> [b14]
  Reinterpret16/1 -> [b15]
  Reinterpret19/1 -> [b16]
  Reinterpret18/1 -> [b17]
  Reinterpret21/1 -> [b18]
  Reinterpret20/1 -> [b19]
  Reinterpret23/1 -> [b20]
  Reinterpret22/1 -> [b21]
  Reinterpret25/1 -> [b22]
  Reinterpret24/1 -> [b23]
  Reinterpret27/1 -> [b24]
  Reinterpret26/1 -> [b25]
  [b0] -> Mult/2
  [b1] -> Mult1/2
  [b2] -> Mult2/2
  [b3] -> Mult3/2
  Delay30/1 -> [we]
  Delay31/1 -> Slice23/1, Slice24/1
  Delay32/1 -> Slice31/1
  Delay33/1 -> Slice32/1
  Delay34/1 -> Slice33/1
  Delay35/1 -> Slice34/1
  Delay36/1 -> Slice35/1
  Delay37/1 -> Slice36/1
  Delay38/1 -> Slice37/1
  Delay39/1 -> Slice38/1
  Delay40/1 -> Slice39/1
  Delay41/1 -> Slice40/1
  Delay42/1 -> Slice41/1
  Delay43/1 -> Slice42/1
  Delay44/1 -> Slice43/1
  Delay29/1 -> Delay14/1, Mult/1
  Slice31/1 -> Single Port RAM2/2
  Slice32/1 -> Single Port RAM3/2
  Slice33/1 -> Single Port RAM4/2
  Slice34/1 -> Single Port RAM1/2
  Slice35/1 -> Single Port RAM5/2
  Slice36/1 -> Single Port RAM6/2
  Slice37/1 -> Single Port RAM7/2
  Slice38/1 -> Single Port RAM8/2
  Slice39/1 -> Single Port RAM9/2
  Slice40/1 -> Single Port RAM10/2
  Slice41/1 -> Single Port RAM11/2
  Slice42/1 -> Single Port RAM12/2
  Slice43/1 -> Single Port RAM13/2
  ? -> ?
  Delay3/1 -> Mult2/1, Delay5/1
  Delay5/1 -> Mult3/1, Delay6/1
  Delay6/1 -> Mult4/1, Delay7/1
  Delay7/1 -> Mult5/1, Delay8/1
  Delay8/1 -> Delay9/1, Mult6/1
  Delay9/1 -> Delay10/1, Mult7/1
  Delay10/1 -> Delay11/1, Mult8/1
  Delay11/1 -> Delay12/1, Mult9/1
  Delay12/1 -> Mult10/1, Delay17/1
  Delay17/1 -> Delay18/1, Mult11/1
  Delay18/1 -> Delay19/1, Mult12/1
  Delay19/1 -> Delay20/1, Mult13/1
  Delay20/1 -> Delay21/1, Mult14/1
  Delay21/1 -> Delay22/1, Mult15/1
  Delay22/1 -> Delay46/1, Mult16/1
  Delay46/1 -> Delay13/1, Mult17/1
  Delay13/1 -> Delay15/1, Mult18/1
  Delay15/1 -> Delay16/1, Mult19/1
  Delay26/1 -> Mult25/1
  Delay16/1 -> Delay1/1, Mult20/1
  Delay1/1 -> Delay2/1, Mult21/1
  Delay2/1 -> Delay4/1, Mult22/1
  Delay4/1 -> Delay25/1, Mult23/1
  Delay25/1 -> Delay26/1, Mult24/1
  Mult/1 -> AddSub25/1
  Mult1/1 -> AddSub25/2
  Mult2/1 -> AddSub1/1
  Mult3/1 -> AddSub1/2
  Mult4/1 -> AddSub2/1
  Mult5/1 -> AddSub2/2
  Mult6/1 -> AddSub3/1
  Mult7/1 -> AddSub3/2
  Mult8/1 -> AddSub4/1
  Mult9/1 -> AddSub4/2
  Mult10/1 -> AddSub7/1
  Mult11/1 -> AddSub7/2
  Mult12/1 -> AddSub5/1
  Mult13/1 -> AddSub5/2
  Mult14/1 -> AddSub6/1
  Mult15/1 -> AddSub6/2
  Mult16/1 -> AddSub8/1
  Mult17/1 -> AddSub8/2
  Mult18/1 -> AddSub9/1
  Mult19/1 -> AddSub9/2
  Mult20/1 -> AddSub10/1
  Mult21/1 -> AddSub10/2
  Mult22/1 -> AddSub11/1
  Mult23/1 -> AddSub11/2
  Mult25/1 -> AddSub12/2
  AddSub11/1 -> AddSub13/1
  AddSub12/1 -> AddSub13/2
  AddSub9/1 -> AddSub14/1
  AddSub10/1 -> AddSub14/2
  AddSub6/1 -> AddSub15/1
  AddSub8/1 -> AddSub15/2
  AddSub7/1 -> AddSub16/1
  AddSub5/1 -> AddSub16/2
  AddSub3/1 -> AddSub17/1
  AddSub4/1 -> AddSub17/2
  AddSub1/1 -> AddSub18/1
  AddSub2/1 -> AddSub18/2
  AddSub25/1 -> Delay27/1
  Delay27/1 -> AddSub19/1
  AddSub18/1 -> AddSub19/2
  AddSub17/1 -> AddSub20/1
  AddSub16/1 -> AddSub20/2
  AddSub15/1 -> AddSub21/1
  AddSub14/1 -> AddSub21/2
  AddSub21/1 -> AddSub22/1
  AddSub13/1 -> Delay28/1
  Delay28/1 -> AddSub22/2
  AddSub19/1 -> AddSub23/2
  AddSub20/1 -> AddSub23/1
  AddSub22/1 -> AddSub40/2
  AddSub23/1 -> AddSub40/1
  AddSub40/1 -> data_out/1

== system chan_snap_v3/LO_SLE ==
  sim_reg : Inport
  chan_snap_v3_LO_SLE_user_data_out : xbsIndex_r4/Gateway In  gui_display_data_type=Fixed-point  arith_type=Unsigned  n_bits=32  bin_pt=0  preci_type=Single  exp_width=8  frac_width=24  quantization="Round  (unbiased: +/- Inf)"  overflow=Saturate  period=1  dbl_ovrd=off  timing_constraint=None  locs_specified=off  LOCs={}  UseAsADC=off  ADCChannel='1'  inherit_from_input=off  hdl_port=on  block_type=gatewayin
  io_delay : xbsIndex_r4/Delay  rst=off  infoeditControl=Selection of Reset will increase slice count due to use of real FFs and instead of SRLs  en=off  latency=0  dbl_ovrd=off  reg_retiming=on  block_type=delay
  reint1 : xbsIndex_r4/Reinterpret  force_arith_type=on  arith_type=Unsigned  force_bin_pt=on  bin_pt=0  block_type=reinterpret
  slice_reg : xbsIndex_r4/Slice  nbits=32  boolean_output=off  mode=Lower Bit Location + Width  bit1=0  base1=MSB of Input  bit0=0  base0=LSB of Input  dbl_ovrd=off  block_type=slice
  in_reg : Outport
  wires:
  chan_snap_v3_LO_SLE_user_data_out/1 -> io_delay/1
  sim_reg/1 -> chan_snap_v3_LO_SLE_user_data_out/1
  io_delay/1 -> slice_reg/1
  slice_reg/1 -> reint1/1
  reint1/1 -> in_reg/1
